simulink model "example1801_2016a"  (Simulink 8.7)
settings: Solver=VariableStepAuto  SolverMode=SingleTasking  StartTime=0.0  StopTime=10.0  RelTol=1e-3
settings Model: Creator=chengqian  LastModifiedBy=chengqian
settings DataIOCC: LimitDataPoints=off  SaveFormat=Dataset
settings DebuggingCC: UnderspecifiedInitializationDetection=Simplified  MergeDetectMultiDrivingBlocksExec=error  SFUnexpectedBacktrackingDiag=error  SFNoUnconditionalDefaultTransitionDiag=error
settings HardwareCC: ProdBitPerPointer=64  ProdLargestAtomicFloat=Float  ProdIntDivRoundTo=Zero  ProdEndianess=LittleEndian  ProdWordSize=64  ProdHWDeviceType=Intel->x86-64 (Windows64)
settings ModelReferenceCC: PropagateSignalLabelsOutOfModel=on
settings SFSimCC: SimUseLocalCustomCode=on
settings RTWCC: RTWUseLocalCustomCode=on
settings GRTTargetCC: TargetLangStandard=C99 (ISO)  GeneratePreprocessorConditionals=Use local settings
settings ConfigComp: CovMetricSettings=dwe  CovHtmlReporting=off  CovSaveCumulativeToWorkspaceVar=off  CovSaveSingleToWorkspaceVar=off  CovModelRefEnable=off  CovExternalEMLEnable=on

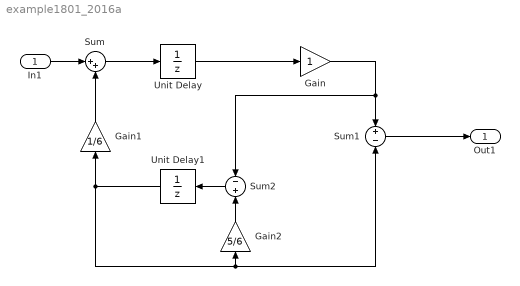
== system example1801_2016a ==
  In1 : Inport
  Gain : Gain
  Gain1 : Gain  Gain=1/6
  Gain2 : Gain  Gain=5/6
  Sum : Sum  Inputs=|++
  Sum1 : Sum  Inputs=+|-
  Sum2 : Sum  Inputs=-|+
  Unit Delay : UnitDelay  SampleTime=-1
  Unit Delay1 : UnitDelay  SampleTime=-1
  Out1 : Outport
  wires:
  In1/1 -> Sum/1
  Sum/1 -> Unit Delay/1
  Unit Delay/1 -> Gain/1
  Gain/1 -> Sum2/1, Sum1/1
  Sum1/1 -> Out1/1
  Gain1/1 -> Sum/2
  Unit Delay1/1 -> Sum1/2, Gain2/1, Gain1/1
  Sum2/1 -> Unit Delay1/1
  Gain2/1 -> Sum2/2
